simulink model "f16_sim"  (Simulink 6.6)
settings: Solver=ode4  StartTime=0.0  StopTime=20  FixedStep=0.02  RelTol=1e-3
values from neighbouring files (symbols this model uses):
  U0TRIM = u0    [f16_init.m]    (also in f16_simulation_loop.m; f16_simulation_turn.m)
settings Model: Creator=joehorn  LastModifiedBy=joehorn
settings DataIOCC: SignalLoggingName=sigsOut
settings DebuggingCC: SignalResolutionControl=TryResolveAllWithWarning  SolverPrmCheckMsg=none  MultiTaskDSMMsg=warning  MultiTaskCondExecSysMsg=none  StrictBusMsg=None
settings HardwareCC: TargetUnknown=on
settings RTWCC: IncludeERTFirstTime=on

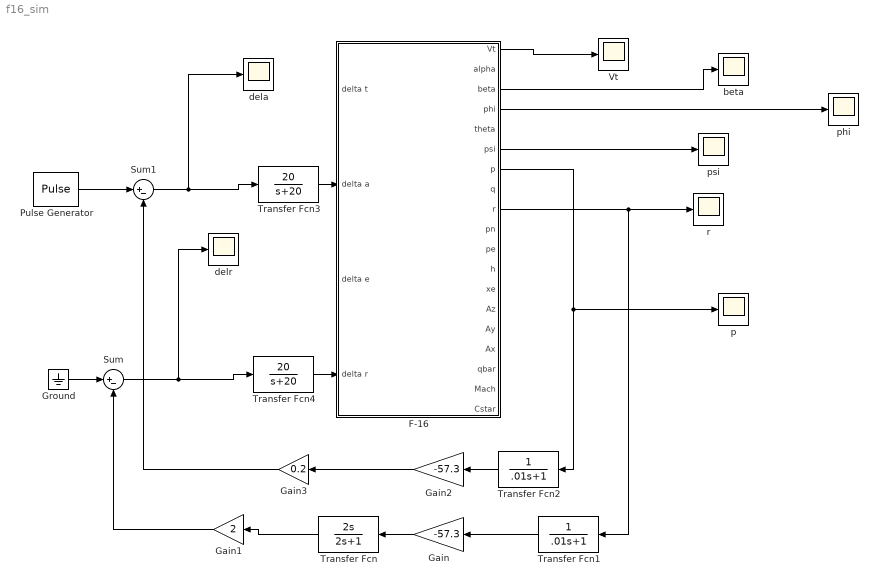
== system f16_sim ==
  F-16 : Subsystem
  Gain : Gain  Orientation=left  Gain=-57.3  SaturateOnIntegerOverflow=on
  Gain1 : Gain  Orientation=left  Gain=2  SaturateOnIntegerOverflow=on
  Gain2 : Gain  Orientation=left  Gain=-57.3  SaturateOnIntegerOverflow=on
  Gain3 : Gain  Orientation=left  Gain=0.2  SaturateOnIntegerOverflow=on
  Ground : Ground
  Pulse Generator : DiscretePulseGenerator  PulseType=Time based  Amplitude=-1  Period=30  PulseWidth=10  PhaseDelay=2
  Sum : Sum  Inputs=|+-  SaturateOnIntegerOverflow=on
  Sum1 : Sum  Inputs=|+-  SaturateOnIntegerOverflow=on
  Transfer Fcn : TransferFcn  Orientation=left  Numerator=[2 0]  Denominator=[2 1]
  Transfer Fcn1 : TransferFcn  Orientation=left  Denominator=[.01 1]
  Transfer Fcn2 : TransferFcn  Orientation=left  Denominator=[.01 1]
  Transfer Fcn3 : TransferFcn  Numerator=20  Denominator=[1 20]
  Transfer Fcn4 : TransferFcn  Numerator=20  Denominator=[1 20]
  Vt : Scope
      settings: YMin=0.05  YMax=0.3
  beta : Scope
      settings: YMin=0  YMax=0.011  SaveName=ScopeData7
  dela : Scope
      settings: YMin=-0.25  YMax=0  SaveName=ScopeData5
  delr : Scope
      settings: YMin=2.77556e-017  YMax=0.5  SaveName=ScopeData2
  p : Scope
      settings: YMin=-0.02  YMax=0.045  SaveName=ScopeData6
  phi : Scope
      settings: YMin=0.1  YMax=0.113  SaveName=ScopeData3
  psi : Scope
      settings: YMin=1.38778e-017  YMax=0.375  SaveName=ScopeData4
  r : Scope
      settings: YMin=0.0032  YMax=0.004
  wires:
  F-16/9(r) -> r/1, Transfer Fcn1/1
  Sum/1 -> delr/1, Transfer Fcn4/1
  F-16/4(phi) -> phi/1
  F-16/6(psi) -> psi/1
  Sum1/1 -> dela/1, Transfer Fcn3/1
  F-16/7(p) -> Transfer Fcn2/1, p/1
  Gain/1 -> Transfer Fcn/1
  Gain2/1 -> Gain3/1
  Transfer Fcn1/1 -> Gain/1
  Transfer Fcn2/1 -> Gain2/1
  Pulse Generator/1 -> Sum1/1
  F-16/1(Vt) -> Vt/1
  Gain1/1 -> Sum/2
  Gain3/1 -> Sum1/2
  F-16/3(beta) -> beta/1
  Transfer Fcn/1 -> Gain1/1
  Transfer Fcn3/1 -> F-16/2(delta a)
  Transfer Fcn4/1 -> F-16/4(delta r)
  Ground/1 -> Sum/1

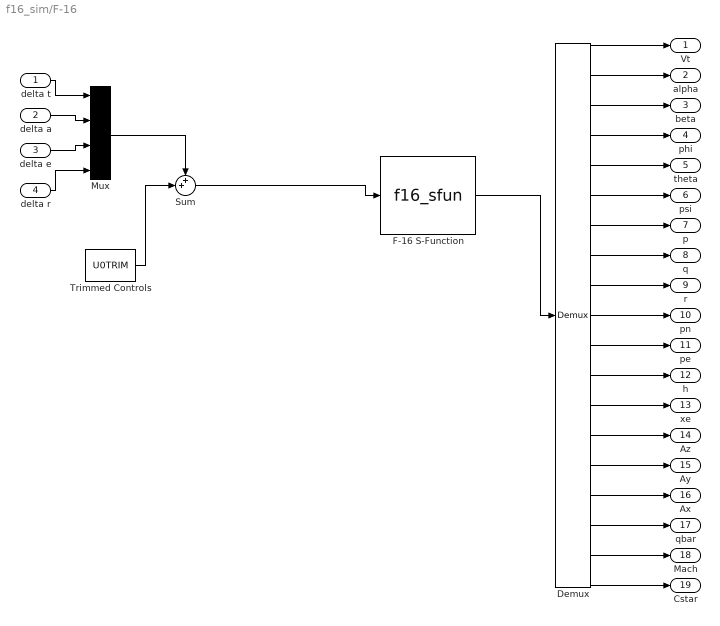
== system f16_sim/F-16 ==
  delta t : Inport
  delta a : Inport  Port=2
  delta e : Inport  Port=3
  delta r : Inport  Port=4
  Demux : Demux  Outputs=19
  F-16 S-Function : S-Function  FunctionName=f16_sfun
  Mux : Mux
  Sum : Sum  Inputs=++|  SaturateOnIntegerOverflow=on
  Trimmed Controls : Constant  Value=U0TRIM
  Vt : Outport
  alpha : Outport  Port=2
  beta : Outport  Port=3
  phi : Outport  Port=4
  theta : Outport  Port=5
  psi : Outport  Port=6
  p : Outport  Port=7
  q : Outport  Port=8
  r : Outport  Port=9
  pn : Outport  Port=10
  pe : Outport  Port=11
  h : Outport  Port=12
  xe : Outport  Port=13
  Az : Outport  Port=14
  Ay : Outport  Port=15
  Ax : Outport  Port=16
  qbar : Outport  Port=17
  Mach : Outport  Port=18
  Cstar : Outport  Port=19
  wires:
  Sum/1 -> F-16 S-Function/1
  Trimmed Controls/1 -> Sum/2
  Mux/1 -> Sum/1
  F-16 S-Function/1 -> Demux/1
  delta t/1 -> Mux/1
  Demux/1 -> Vt/1
  delta a/1 -> Mux/2
  delta e/1 -> Mux/3
  delta r/1 -> Mux/4
  Demux/16 -> Ax/1
  Demux/17 -> qbar/1
  Demux/18 -> Mach/1
  Demux/2 -> alpha/1
  Demux/3 -> beta/1
  Demux/4 -> phi/1
  Demux/5 -> theta/1
  Demux/6 -> psi/1
  Demux/7 -> p/1
  Demux/8 -> q/1
  Demux/9 -> r/1
  Demux/10 -> pn/1
  Demux/11 -> pe/1
  Demux/12 -> h/1
  Demux/13 -> xe/1
  Demux/14 -> Az/1
  Demux/15 -> Ay/1
  Demux/19 -> Cstar/1
